simulink model "stm32test"  (R2024b)
settings: Solver=FixedStepAuto  StartTime=0.0  StopTime=inf  RelTol=1e-3  EnableMultiTasking=on
libraries: stm32f4xxblockslib x17, simulink x14, dspstat3 x2, stm32blockslib x2, simulink_extras x2, Blokk_Konyvtar x1
settings Model: STM32="{\"DigitalPortRead\":[{\"ID\":\"stm32test:431\"},{\"ID\":\"stm32test:432\"},{\"ID\":\"stm32test:483\"},{\"ID\":\"stm32test:484\"},{\"ID\":\"stm32test:504\"},{\"ID\":\"stm32test:505\"},{\"ID\":\"stm32test:895\"},{\"ID\":\"stm32test:896\"},{\"ID\":\"stm32test:1060\"},{\"ID\":\"stm32test:1031\"},{\"ID\":\"stm32test:1185\"},{\"ID\":\"stm32test:1186\"},{\"ID\":\"stm32test:1192\"},{\"ID\":\"stm32test:1193\"},{\"ID\":\"stm32test:1194\"},{\"ID\":\"stm32test:1195\"},{\"ID\":\"stm32test:1388:438\"},{\"ID\":\"stm32test:1424\"},{\"ID\":\"stm32test:1590\"}],\"PWMOutput\":[{\"ID\":\"stm32test:6\"},{\"ID\":\"stm32test:8\"},{\"ID\":\"stm32test:1305\"},{\"ID\":\"stm32test:1306\"},{\"ID\":\"stm32test:1562\"}],\"DigitalPortWrite\":[{\"ID\":\"stm32test:1295\"},{\"ID\":\"stm32test:1307\"},{\"ID\":\"stm32test:1481\"},{\"ID\":\"stm32test:1482\"}],\"TimerCapture\":[{\"ID\":\"stm32test:166\"},{\"ID\":\"stm32test:836\"},{\"ID\":\"stm32test:1074\"},{\"ID\":\"stm32test:1045\"},{\"ID\":\"stm32test:1103\"},{\"ID\":\"stm32test:1388:414\"},{\"ID\":\"stm32test:1132\"},{\"ID\":\"stm32test:1468:414\"},{\"ID\":\"stm32test:1542\"}],\"HardwareInterrupt\":[{\"ID\":\"stm32test:102\"},{\"ID\":\"stm32test:1388:418\"}]}"  Creator=Tarsoly  LastModifiedBy=Asus
settings OptimizationCC: BlockReduction=off  BooleanDataType=off  EnhancedBackFolding=on  PassReuseOutputArgsAs=Individual arguments  ZeroExternalMemoryAtStartup=off  ZeroInternalMemoryAtStartup=off  MaxStackSize=512  OptimizeBlockOrder=speed  DifferentSizesBufferReuse=on  OptimizationCustomize=off  EfficientTunableParamExpr=on
settings DebuggingCC: SaveWithParameterizedLinksMsg=none  MergeDetectMultiDrivingBlocksExec=none  SignalResolutionControl=TryResolveAllWithWarning  ParameterTunabilityLossMsg=error
settings HardwareCC: ProdBitPerPointer=32  ProdBitPerSizeT=32  ProdBitPerPtrDiffT=32  ProdLargestAtomicInteger=Long  ProdLargestAtomicFloat=Double  ProdWordSize=32  ProdHWDeviceType=ARM Compatible->ARM Cortex-M  TargetLargestAtomicInteger=Long  TargetLargestAtomicFloat=Double  TargetIntDivRoundTo=Zero  TargetEndianess=LittleEndian  TargetHWDeviceType=ARM Compatible->ARM Cortex-M
settings ModelReferenceCC: PropagateSignalLabelsOutOfModel=off
settings SFSimCC: SimCustomHeaderCode="#include \"SensorActuator.h\""  SimCustomInitializer=Timer_Init_Custom();  SimUserSources=SensorActuator.c  SimUserDefines=STM32F411xE  MATLABDynamicMemAlloc=off
settings SFSimCC: SimUserIncludeDirs=|
  | D:\BME\Hetedik_felev\Szakdoga\Matlab\C_kod
  | D:\CubeMXProjectFiles\tanfolyamrobot\Core\Inc
  | D:\CubeMXProjectFiles\tanfolyamrobot\Drivers\STM32F4xx_HAL_Driver\Inc
  | D:\CubeMXProjectFiles\tanfolyamrobot\Drivers\CMSIS\Device\ST\STM32F4xx\Include
  | D:\CubeMXProjectFiles\tanfolyamrobot\Drivers\CMSIS\Include
settings RTWCC: Description=Embedded Coder  SystemTargetFile=ert.tlc  HardwareBoard=STM32F4xx Based  TemplateMakefile=ert_default_tmf  RTWUseSimCustomCode=on  CustomHeaderCode="#include \"SensorActuator.h\""  CustomSource=SensorActuator.c  CustomDefine=STM32F411xE  CustomInitializer=Timer_Init_Custom();  Toolchain=GNU Tools for ARM Embedded Processors
settings RTWCC: CustomInclude=|
  | D:\BME\Hetedik_felev\Szakdoga\Matlab\C_kod
  | D:\CubeMXProjectFiles\tanfolyamrobot\Core\Inc
  | D:\CubeMXProjectFiles\tanfolyamrobot\Drivers\STM32F4xx_HAL_Driver\Inc
  | D:\CubeMXProjectFiles\tanfolyamrobot\Drivers\CMSIS\Device\ST\STM32F4xx\Include
  | D:\CubeMXProjectFiles\tanfolyamrobot\Drivers\CMSIS\Include
settings CodeAppCC: ForceParamTrailComments=on  IgnoreCustomStorageClasses=off  OperatorAnnotations=on  SimulinkDataObjDesc=on  SFDataObjDesc=on  InsertBlockDesc=on
settings ERTTargetCC: TargetLangStandard=C99 (ISO)  CodeReplacementLibrary=ARM Cortex-M  ExtModeTransport=3  ExtModeStaticAlloc=on  ExtModeStaticAllocSize=2048  ExtModeMexFile=ext_xcp  ExtModeIntrfLevel=Level2 - Open  InlinedParameterPlacement=Hierarchical

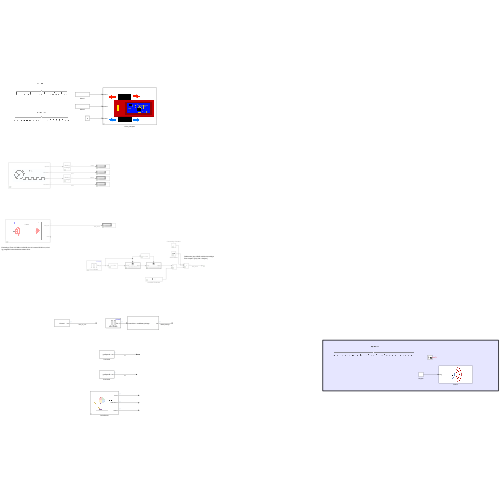
[thumbnail: Simulink's stored preview of the top-level diagram]
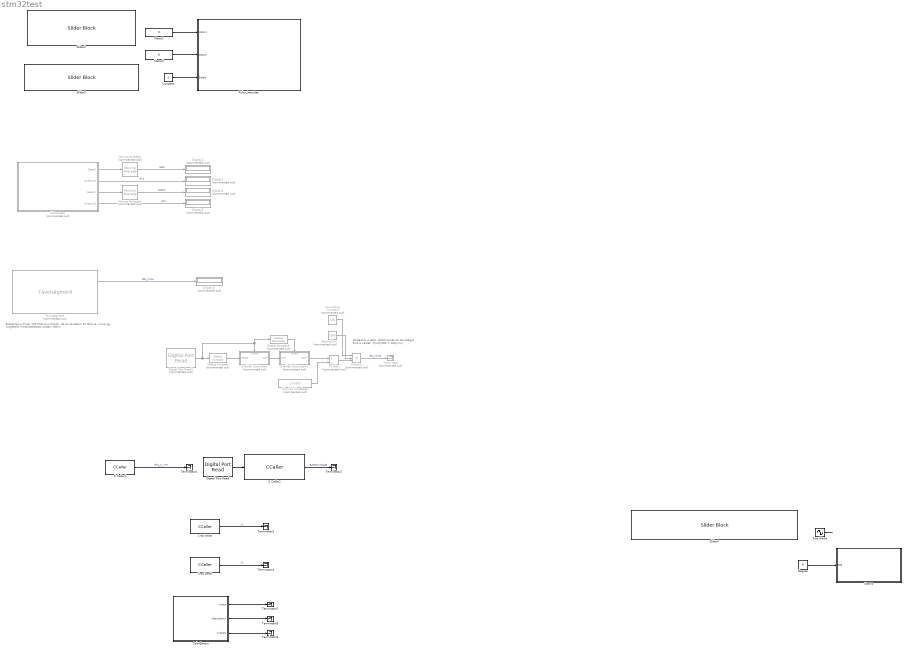
== system stm32test ==
  note: Eredetileg a Timer 100 MHz-el működik, de én levettem 25 MHz-re, mivel
      | így megfelelő mintavételezést tudtam elérni.
  note: Skálázzuk a jelet, időből csinálunk távolságot
      | Erra a képlet: T[ms]*100 = dist[mm]
  1-es kerek : CCaller  FunctionName=getSpeedA  PortSpecificationStruct="%)30     .    & (   8    (     @         %    \"     $    !     0         %  0 \"0    $    _    07)G3F%M90  4&]R=$YA;64 4V-O<&4     26YD97@     5'EP90      4VEZ90      27-';&]B86P   X    P    !@    @    $          4    (     0    ,    !         !   P!O=70 #@   #     &    \"     0         !0    @    !     P    $         $  # &]U=  .    .     8    (    !          %    \"     $    &     0         0    !@   $]U='!U=   #@   #@    &    \"     8         !0    @    !     0    $         \"0    @               X    X    !@    @    $          4    (     0    8    !         !     &    9&]U8FQE   .    ,     8    (    !          %    \"     $    !     0         0  $ ,0    X    P    !@    @    ) @        4    (     0    $    !          (  0"  SampleTime=0.02
  2-es kerek : CCaller  FunctionName=getSpeedB  PortSpecificationStruct="%)30     .    & (   8    (     @         %    \"     $    !     0         %  0 \"0    $    _    07)G3F%M90  4&]R=$YA;64 4V-O<&4     26YD97@     5'EP90      4VEZ90      27-';&]B86P   X    P    !@    @    $          4    (     0    ,    !         !   P!O=70 #@   #     &    \"     0         !0    @    !     P    $         $  # &]U=  .    .     8    (    !          %    \"     $    &     0         0    !@   $]U='!U=   #@   #@    &    \"     8         !0    @    !     0    $         \"0    @               X    X    !@    @    $          4    (     0    8    !         !     &    9&]U8FQE   .    ,     8    (    !          %    \"     $    !     0         0  $ ,0    X    P    !@    @    ) @        4    (     0    $    !          (  0"  SampleTime=0.02
  C Caller1 : CCaller  FunctionName=infrared  PortSpecificationStruct="%)30     .    & (   8    (     @         %    \"     $    !     0         %  0 \"0    $    _    07)G3F%M90  4&]R=$YA;64 4V-O<&4     26YD97@     5'EP90      4VEZ90      27-';&]B86P   X    P    !@    @    $          4    (     0    ,    !         !   P!O=70 #@   #     &    \"     0         !0    @    !     P    $         $  # &]U=  .    .     8    (    !          %    \"     $    &     0         0    !@   $]U='!U=   #@   #@    &    \"     8         !0    @    !     0    $         \"0    @               X    X    !@    @    $          4    (     0    8    !         !     &    =6EN=#,R   .    ,     8    (    !          %    \"     $    !     0         0  $ ,0    X    P    !@    @    ) @        4    (     0    $    !          (  0"  SampleTime=0.02
  C Caller2 : CCaller  FunctionName=readBatteryVoltage  PortSpecificationStruct="%)30     .    V ,   8    (     @         %    \"     (    !     0         %  0 \"0    $    _    07)G3F%M90  4&]R=$YA;64 4V-O<&4     26YD97@     5'EP90      4VEZ90      27-';&]B86P   X    P    !@    @    $          4    (     0    ,    !         !   P!O=70 #@   #     &    \"     0         !0    @    !     P    $         $  # &]U=  .    .     8    (    !          %    \"     $    &     0         0    !@   $]U='!U=   #@   #@    &    \"     8         !0    @    !     0    $         \"0    @               X    X    !@    @    $          4    (     0    8    !         !     &    =6EN=#$V   .    ,     8    (    !          %    \"     $    !     0         0  $ ,0    X    P    !@    @    ) @        4    (     0    $    !          (  0      #@   $     &    \"     0         !0    @    !    \"P    $         $     L   !B=71T;VY686QU90      #@   $     &    \"     0         !0    @    !    \"P    $         $     L   !B=71T;VY686QU90      #@   #@    &    \"     0         !0    @    !    !0    $         $     4   !);G!U=     X    X    !@    @    &          4    (     0    $    !          D    (               .    .     8    (    !          %    \"     $    '     0         0    !P   &)O;VQE86X #@   #     &    \"     0         !0    @    !     0    $         $  ! #$    .    ,     8    (    \"0(        %    \"     $    !     0         \"  $"  SampleTime=1
  ColorSensor : Subsystem
      mask DialogControl DescTextVar Prompt: This subsystem is for measuring the color of the ground beneath the robot.
      mask Display: image('Mask5_szin2.png', [20,20,20,20,100,100]);
  Constant : Constant
  Converting Constant : Constant  Commented=on  Value=100
  Degree : Constant  Value=0
  Detect Decrease : simulink/Logic and Bit Operations/Detect Decrease  Commented=on  vinit=0.0  OutDataTypeStr=boolean
  Detect Increase : simulink/Logic and Bit Operations/Detect Increase  Commented=on  vinit=0.0  OutDataTypeStr=boolean
  Digital Port Read : stm32f4xxblockslib/Digital Port Read  PortName=GPIOA  PinNumber=[15]  ReadOperation=on  IOAsArray=off  SampleTime=1  EnableSimPort=off  hoistedMaskSrc=ECSoC/ECSimCodegen/Digital Port Read
  Digital Port Read1 : stm32f4xxblockslib/Digital Port Read  Commented=on  PortName=GPIOB  PinNumber=[7]  ReadOperation=on  IOAsArray=on  SampleTime=0.0001  EnableSimPort=off  hoistedMaskSrc=ECSoC/ECSimCodegen/Digital Port Read
  Display{1..4,6} (5 alike) : Display  Commented=on
  Divide1 : Product  Commented=on  Inputs=*/
  Enabled Subsystem : Subsystem  Commented=on  TreatAsAtomicUnit=on
  Enabled Subsystem1 : Subsystem  Commented=on  TreatAsAtomicUnit=on
  Kulon_iranyitas : Subsystem
      mask DialogControl Control2 Prompt: This block is meant for when you want to control the wheels independent of eachother. It can control the wheels with (-99;99) signals.
      mask Display: image('Maszk4_kulon_kerek.png', [25,25,5,0,100,100]);
  Motor1 : Constant  Value=0
  Motor2 : Constant  Value=0
  Moving Average : dspstat3/Moving Average  Commented=on  Method=Sliding window  ForgettingFactorPort=off  SpecifyWindowLength=on  WindowLength=5  OverlapLength=4  AllowArbitraryInputLength=off  ForgettingFactor=0.9  SimulateUsing=Interpreted execution
  Moving Average1 : dspstat3/Moving Average  Commented=on  Method=Sliding window  ForgettingFactorPort=off  SpecifyWindowLength=on  WindowLength=9  OverlapLength=8  AllowArbitraryInputLength=off  ForgettingFactor=0.9  SimulateUsing=Interpreted execution
  Product : Product  Commented=on  Inputs=3
  Second2ms : Constant  Commented=on  Value=1000
  Simulink Timebase : Constant  Commented=on  Value=1/0.0001
  Sine Wave : Sin  Amplitude=90  Frequency=pi  SampleTime=0.02
  Slider2 : SliderBlock  ScaleMin=-99  ScaleMax=99
  Slider3 : SliderBlock  ScaleMin=-99  ScaleMax=99
  Slider4 : SliderBlock  ScaleMin=-90  ScaleMax=90
  Subsystem : Subsystem  Commented=on  mask{TimClkFrq=25e6, CPR=1024, fwdvalue1=0, fwdvalue2=1, bckvalue1=1, bckvalue2=0, PrScaler=1}
      mask prompts: TimClkFrq "Timer Clock Frequency"; CPR "Counts Per Revolution"; fwdvalue1 "Forward Direction Value 1"; fwdvalue2 "Forward Direction Value 2"; bckvalue1 "Backward Direction Value 1"; bckvalue2 "Backward Direction Value 2"; PrScaler "Timer Prescaler (Shouldn't be Zero)"
      mask DialogControl DescTextVar Prompt: This block takes the encoder signal and converts it into speed and direction. The frequency of the timer channel and the counts per revolution is required to be filled with the correct values. The direction signals for each wheel is also customisable, thus the wheels may have a different base direction. The block uses Timer5 hardware interrupt on all 4 channels and reads PA0-3 GPIO ports. Modifying this requires looking under the mask.
      mask Display: image('Mask1.png', [30,10,30,10,100,100]);
  Szervo : Subsystem
      mask Display: image('Mask6_Szervo.png', [30,10,30,10,100,100]);
  Terminator : Terminator  Commented=on
  Terminator{1..7} (7 alike) : Terminator
  Távolságmérő : Blokk_Konyvtar/Távolságmérő  Commented=on  TimClkFrq=25e6  PrScaler=15000  OoR_const=2000
      settings: SourceProductName=Blokk_Konyvtar
  wires:
  Moving Average/1 -> Display2/1  "rad/s"
  Moving Average1/1 -> Display4/1  "rad/s2"
  Távolságmérő/1 -> Display6/1  "dist_mma"
  Subsystem/1(Speed1) -> Moving Average/1
  Subsystem/2(Direction1) -> Display1/1  "dir1"
  Subsystem/3(Speed 2) -> Moving Average1/1
  Subsystem/4(Direction2) -> Display3/1  "dir2"
  Constant/1 -> Kulon_iranyitas/3(Enable)
  Motor1/1 -> Kulon_iranyitas/1(Motor1)
  Motor2/1 -> Kulon_iranyitas/2(Motor2)
  Digital Port Read1/1 -> Detect Increase/1, Detect Decrease/1, Enabled Subsystem/Enable
  Detect Increase/1 -> Enabled Subsystem/1(Reset)
  Enabled Subsystem/1(CNT) -> Enabled Subsystem1/1(CNT)
  Detect Decrease/1 -> Enabled Subsystem1/Enable
  Second2ms/1 -> Product/2
  Enabled Subsystem1/1(Latch) -> Divide1/1
  Converting Constant/1 -> Product/1
  Simulink Timebase/1 -> Divide1/2
  Divide1/1 -> Product/3
  Product/1 -> Terminator/1  "dist_mmb"
  C Caller1/1 -> Terminator1/1  "Infra_C_mm"
  C Caller2/1 -> Terminator2/1  "BatteryVoltage"
  Digital Port Read/1 -> C Caller2/1
  2-es kerek/1 -> Terminator4/1  "v2"
  1-es kerek/1 -> Terminator3/1  "v1"
  Sine Wave/1 -> ?
  ColorSensor/1(<Hue>) -> Terminator7/1
  ColorSensor/2(<Saturation>) -> Terminator5/1
  ColorSensor/3(<Value>) -> Terminator6/1
  Degree/1 -> Szervo/1(Deg)

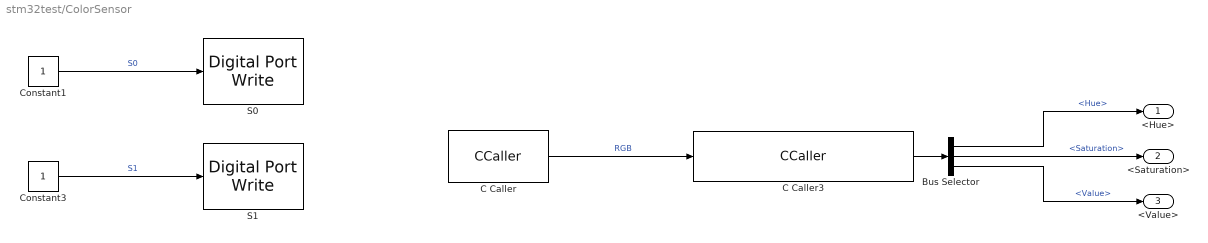
== system stm32test/ColorSensor ==
  Bus Selector : BusSelector  OutputSignals=Hue,Saturation,Value
  C Caller : CCaller  FunctionName=getRGB  PortSpecificationStruct="%)30     .    ( (   8    (     @         %    \"     $    !     0         %  0 \"0    $    _    07)G3F%M90  4&]R=$YA;64 4V-O<&4     26YD97@     5'EP90      4VEZ90      27-';&]B86P   X    P    !@    @    $          4    (     0    ,    !         !   P!O=70 #@   #     &    \"     0         !0    @    !     P    $         $  # &]U=  .    .     8    (    !          %    \"     $    &     0         0    !@   $]U='!U=   #@   #@    &    \"     8         !0    @    !     0    $         \"0    @               X   !     !@    @    $          4    (     0    H    !         !     *    0G5S.B!21T)?=         X    P    !@    @    $          4    (     0    $    !         !   0 Q    #@   #     &    \"     D\"        !0    @    !     0    $          @ !"  SampleTime=0.02
  C Caller3 : CCaller  FunctionName=getHSVfromRGB  PortSpecificationStruct="%)30     .    Z ,   8    (     @         %    \"     (    !     0         %  0 \"0    $    _    07)G3F%M90  4&]R=$YA;64 4V-O<&4     26YD97@     5'EP90      4VEZ90      27-';&]B86P   X    P    !@    @    $          4    (     0    ,    !         !   P!O=70 #@   #     &    \"     0         !0    @    !     P    $         $  # &]U=  .    .     8    (    !          %    \"     $    &     0         0    !@   $]U='!U=   #@   #@    &    \"     8         !0    @    !     0    $         \"0    @               X   !     !@    @    $          4    (     0    H    !         !     *    0G5S.B!(4U9?=         X    P    !@    @    $          4    (     0    $    !         !   0 Q    #@   #     &    \"     D\"        !0    @    !     0    $          @ !       .    0     8    (    !          %    \"     $    +     0         0    \"P   &UE87-U<F5M96YT       .    0     8    (    !          %    \"     $    +     0         0    \"P   &UE87-U<F5M96YT       .    .     8    (    !          %    \"     $    %     0         0    !0   $EN<'5T    #@   #@    &    \"     8         !0    @    !     0    $         \"0    @               X   !     !@    @    $          4    (     0    H    !         !     *    0G5S.B!21T)?=         X    P    !@    @    $          4    (     0    $    !         !   0 Q    #@   #     &    \"     D\"        !0    @    !     0    $          @ !"
  Constant1 : Constant
  Constant3 : Constant
  S0 : stm32f4xxblockslib/Digital Port Write  PortName=GPIOC  PinNumber=[12]  ReadOperation=off  IOAsArray=on  EnableSimPort=off  hoistedMaskSrc=ECSoC/ECSimCodegen/Digital Port Write
  S1 : stm32f4xxblockslib/Digital Port Write  PortName=GPIOD  PinNumber=[2]  ReadOperation=off  IOAsArray=on  EnableSimPort=off  hoistedMaskSrc=ECSoC/ECSimCodegen/Digital Port Write
  <Hue> : Outport
  <Saturation> : Outport  Port=2
  <Value> : Outport  Port=3
  wires:
  C Caller/1 -> C Caller3/1  "RGB"
  Constant3/1 -> S1/1  "S1"
  Bus Selector/3 -> <Value>/1  "<Value>"
  C Caller3/1 -> Bus Selector/1
  Constant1/1 -> S0/1  "S0"
  Bus Selector/2 -> <Saturation>/1  "<Saturation>"
  Bus Selector/1 -> <Hue>/1  "<Hue>"

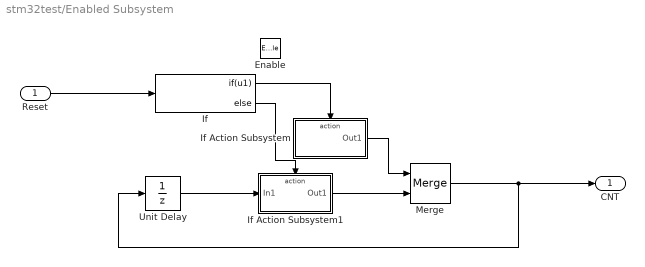
== system stm32test/Enabled Subsystem ==
  Reset : Inport
  Enable : EnablePort
  If : If  IfExpression=u1
  If Action Subsystem : Subsystem  TreatAsAtomicUnit=on
  If Action Subsystem1 : Subsystem  TreatAsAtomicUnit=on
  Merge : Merge
  Unit Delay : UnitDelay  SampleTime=-1  HasFrameUpgradeWarning=on
  CNT : Outport
  wires:
  Merge/1 -> Unit Delay/1, CNT/1
  Reset/1 -> If/1
  If/1 -> If Action Subsystem/Action
  If Action Subsystem/1(Out1) -> Merge/1
  If/2 -> If Action Subsystem1/Action
  If Action Subsystem1/1(Out1) -> Merge/2
  Unit Delay/1 -> If Action Subsystem1/1(In1)

== system stm32test/Enabled Subsystem1 ==
  CNT : Inport
  Enable : EnablePort
  Latch : Outport
  wires:
  CNT/1 -> Latch/1

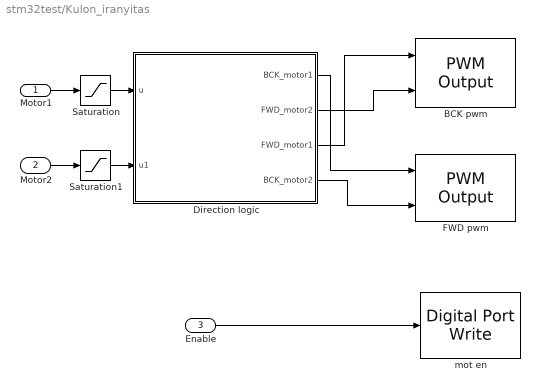
== system stm32test/Kulon_iranyitas ==
  Motor1 : Inport
  Motor2 : Inport  Port=2
  Enable : Inport  Port=3
  BCK pwm : stm32f4xxblockslib/PWM Output  TimerModule=TIM1  DutycycleUnits=Percentage  EnableChannel1=on  EnableChannel2=on  EnableChannel3=off  EnableChannel4=off  EnableCounterInput=off  EnableMainOutputInput=off  EnableFrequencyInput=off  SetRCAfterCE=off  OutputDirection=off  OutputMainOutputEnableStatus=off  SampleTime=0.1  EnableSimPort=off  EnableUpdateEvent=off  EnableCaptureCompare1Event=off  EnableCaptureCompare2Event=off  EnableCaptureCompare3Event=off  EnableCaptureCompare4Event=off  EnableTriggerEvent=off  EnableBreakEvent=off  ProcessorFamily=STM32F4  hoistedMaskSrc=ECSoC/ECSimCodegen/PWM Output
  Direction logic : Subsystem
  "FWD pwm " : stm32f4xxblockslib/PWM Output  TimerModule=TIM3  DutycycleUnits=Percentage  EnableChannel1=off  EnableChannel2=off  EnableChannel3=on  EnableChannel4=on  EnableCounterInput=off  EnableMainOutputInput=off  EnableFrequencyInput=off  SetRCAfterCE=off  OutputDirection=off  OutputMainOutputEnableStatus=off  SampleTime=0.1  EnableSimPort=off  EnableUpdateEvent=off  EnableCaptureCompare1Event=off  EnableCaptureCompare2Event=off  EnableCaptureCompare3Event=off  EnableCaptureCompare4Event=off  EnableTriggerEvent=off  EnableBreakEvent=off  ProcessorFamily=STM32F4  hoistedMaskSrc=ECSoC/ECSimCodegen/PWM Output
  Saturation : Saturate  UpperLimit=99  LowerLimit=-99
  Saturation1 : Saturate  UpperLimit=99  LowerLimit=-99
  mot en : stm32f4xxblockslib/Digital Port Write  PortName=GPIOC  PinNumber=5  ReadOperation=off  IOAsArray=on  EnableSimPort=off  hoistedMaskSrc=ECSoC/ECSimCodegen/Digital Port Write
  wires:
  Enable/1 -> mot en/1
  Motor1/1 -> Saturation/1
  Motor2/1 -> Saturation1/1
  Direction logic/1(BCK_motor1) -> "FWD pwm "/1
  Direction logic/2(FWD_motor2) -> BCK pwm/2
  Direction logic/3(FWD_motor1) -> BCK pwm/1
  Direction logic/4(BCK_motor2) -> "FWD pwm "/2
  Saturation/1 -> Direction logic/1(u)
  Saturation1/1 -> Direction logic/2(u1)

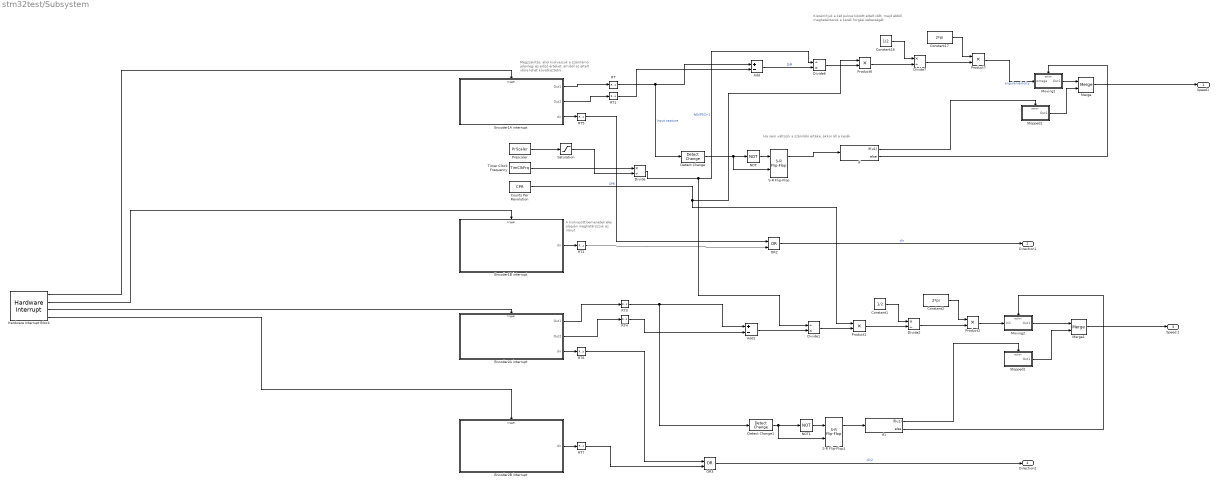
== system stm32test/Subsystem ==
  note: Kiszámítjuk a két pulzus között eltelt időt, majd ebből meghatározzuk a kerék forgási sebességét
  note: Ha nem változik a számláló értéke, akkor áll a kerék
  note: A kiolvasott bemenetek élei alapján meghatározzuk az irányt
  note: Megszakítás, ahol kiolvassuk a számlámó jelenlegi és előző értéket, amiből az eltelt időre lehet következtetni
  Add : Sum  Inputs=+-
  Add1 : Sum  Inputs=+-
  Constant1 : Constant  Value=1/2
  Constant16 : Constant  Value=1/2
  Constant17 : Constant  Value=2*pi
  Constant2 : Constant  Value=2*pi
  Counts Per Revolution : Constant  Value=CPR
  Detect Change : simulink/Logic and Bit Operations/Detect Change  vinit=0  OutDataTypeStr=boolean
      settings: LibrarySourceBlock=|
      | hdlsllib/Logic and Bit
      | Operations/Detect
      | Change
  Detect Change1 : simulink/Logic and Bit Operations/Detect Change  vinit=0  OutDataTypeStr=boolean
      settings: LibrarySourceBlock=|
      | hdlsllib/Logic and Bit
      | Operations/Detect
      | Change
  Divide : Product  Inputs=*/
  Divide1 : Product  Inputs=/*
  Divide2 : Product  Inputs=*/
  Divide6 : Product  Inputs=/*
  Divide7 : Product  Inputs=*/
  Encoder1A interrupt : Subsystem  TreatAsAtomicUnit=on
  Encoder1B interrupt : Subsystem  TreatAsAtomicUnit=on
  Encoder2A interrupt : Subsystem  TreatAsAtomicUnit=on
  Encoder2B interrupt : Subsystem  TreatAsAtomicUnit=on
  Hardware Interrupt Block : stm32f4xxblockslib/Hardware Interrupt  ISRGroup=Timer (TIM)  ISRName=TIM5_IRQHandler  ISRNumber=65  EventsList={ 'off', 'TIM5 Update', '1'; 'on', 'TIM5 CC1', '2'; 'on', 'TIM5 CC2', '3'; 'on', 'TIM5 CC3', '4'; 'on', 'TIM5 CC4', '5'; 'off', 'TIM5 Trigger', '6'; 'off', 'Custom event', '7' }  SelectedEvents={'TIM5 CC1','TIM5 CC2','TIM5 CC3','TIM5 CC4'}  TaskPriority=30  DisablePreemption=off  ClearInterruptFlagsAtEndOfEvent=on  InterruptDefinitionFile=$(TARGET_ROOT)/registry/interrupts/STM32F4xxBased_interrupts.xml  HardwareBoard=STM32F4xx Based  EnableSimPort=off
  If : If  IfExpression=u1
  If1 : If  IfExpression=u1
  Merge : Merge
  Merge1 : Merge
  Moving1 : Subsystem  TreatAsAtomicUnit=on
  Moving2 : Subsystem  TreatAsAtomicUnit=on
  NOT : Logic  Operator=NOT  IconShape=distinctive  AllPortsSameDT=off  OutDataTypeStr=boolean
  NOT1 : Logic  Operator=NOT  IconShape=distinctive  AllPortsSameDT=off  OutDataTypeStr=boolean
  OR2 : Logic  Operator=OR  IconShape=distinctive  AllPortsSameDT=off  OutDataTypeStr=boolean
  OR3 : Logic  Operator=OR  IconShape=distinctive  AllPortsSameDT=off  OutDataTypeStr=boolean
  Prescaler : Constant  Value=PrScaler
  Product{1..2,6..7} (4 alike) : Product
  RT{,1..7} (8 alike) : RateTransition  Deterministic=off  OutPortSampleTime=0.02
  S-R Flip-Flop : simulink_extras/Flip Flops/S-R Flip-Flop  initial_condition=0
  S-R Flip-Flop1 : simulink_extras/Flip Flops/S-R Flip-Flop  initial_condition=0
  Saturation : Saturate  UpperLimit=inf  LowerLimit=1
  Stopped1 : Subsystem  TreatAsAtomicUnit=on
  Stopped2 : Subsystem  TreatAsAtomicUnit=on
  Timer Clock Frequency : Constant  Value=TimClkFrq
  Speed1 : Outport
  Direction1 : Outport  Port=2
  Speed 2 : Outport  Port=3
  Direction2 : Outport  Port=4
  wires:
  S-R Flip-Flop1/1 -> If1/1
  Hardware Interrupt Block/4 -> Encoder2B interrupt/Trigger
  Encoder1A interrupt/2(Out2) -> RT1/1
  Product7/1 -> Moving1/1(omega)  "angularvelocity"
  Stopped2/1(Out1) -> Merge1/2
  If/1 -> Stopped1/Action
  Moving1/1(Out1) -> Merge/1
  RT6/1 -> OR3/1
  If/2 -> Moving1/Action
  Hardware Interrupt Block/2 -> Encoder1B interrupt/Trigger
  Detect Change1/1 -> NOT1/1, S-R Flip-Flop1/2
  Hardware Interrupt Block/1 -> Encoder1A interrupt/Trigger
  Encoder2A interrupt/1(Out1) -> RT3/1
  If1/1 -> Stopped2/Action
  OR3/1 -> Direction2/1  "dir2"
  NOT/1 -> S-R Flip-Flop/1
  RT4/1 -> Add1/2
  Encoder2A interrupt/2(Out2) -> RT4/1
  Encoder1A interrupt/1(Out1) -> RT/1
  S-R Flip-Flop/1 -> If/1
  RT7/1 -> OR3/2
  Moving2/1(Out1) -> Merge1/1
  Hardware Interrupt Block/3 -> Encoder2A interrupt/Trigger
  If1/2 -> Moving2/Action
  RT/1 -> Add/1, Detect Change/1  "Input capture"
  Stopped1/1(Out1) -> Merge/2
  RT3/1 -> Add1/1, Detect Change1/1
  RT5/1 -> OR2/1
  RT2/1 -> OR2/2
  NOT1/1 -> S-R Flip-Flop1/1
  Merge1/1 -> Speed 2/1
  Detect Change/1 -> NOT/1, S-R Flip-Flop/2
  Merge/1 -> Speed1/1
  RT1/1 -> Add/2
  Product2/1 -> Moving2/1(In1)
  OR2/1 -> Direction1/1  "dir"
  Encoder1B interrupt/1(dir) -> RT2/1
  Encoder1A interrupt/3(dir) -> RT5/1
  Encoder2A interrupt/3(dir) -> RT6/1
  Encoder2B interrupt/1(dir) -> RT7/1
  Timer Clock Frequency/1 -> Divide/1
  Prescaler/1 -> Saturation/1
  Divide/1 -> Divide6/1, Divide1/1  "fclk/PSC+1"
  Counts Per Revolution/1 -> Product1/1, Product6/1  "CPR"
  Product6/1 -> Divide7/2
  Divide7/1 -> Product7/2
  Divide6/1 -> Product6/2
  Add/1 -> Divide6/2  "Diff"
  Constant17/1 -> Product7/1
  Constant16/1 -> Divide7/1
  Saturation/1 -> Divide/2
  Divide1/1 -> Product1/2
  Add1/1 -> Divide1/2
  Constant1/1 -> Divide2/1
  Product1/1 -> Divide2/2
  Divide2/1 -> Product2/2
  Constant2/1 -> Product2/1

== system stm32test/Szervo ==
  Deg : Inport
  PWM Output : stm32f4xxblockslib/PWM Output  TimerModule=TIM11  DutycycleUnits=Percentage  EnableChannel1=on  EnableChannel2=off  EnableChannel3=off  EnableChannel4=off  EnableCounterInput=off  EnableMainOutputInput=off  EnableFrequencyInput=off  SetRCAfterCE=off  OutputDirection=off  OutputMainOutputEnableStatus=off  SampleTime=0.1  EnableSimPort=off  EnableUpdateEvent=off  EnableCaptureCompare1Event=off  EnableCaptureCompare2Event=off  EnableCaptureCompare3Event=off  EnableCaptureCompare4Event=off  EnableTriggerEvent=off  EnableBreakEvent=off  ProcessorFamily=STM32F4  hoistedMaskSrc=ECSoC/ECSimCodegen/PWM Output
  Subsystem2 : Subsystem
  wires:
  Subsystem2/1(f(x)) -> PWM Output/1  "percent"
  Deg/1 -> Subsystem2/1(x)  "x"

== system stm32test/Enabled Subsystem/If Action Subsystem ==
  Action Port : ActionPort  ActionPortLabel=if(u1)
  Constant : Constant  Value=0
  Out1 : Outport
  wires:
  Constant/1 -> Out1/1

== system stm32test/Enabled Subsystem/If Action Subsystem1 ==
  In1 : Inport
  Action Port : ActionPort  ActionPortLabel=else
  Add Constant : Bias  Bias=1  SaturateOnIntegerOverflow=off
  Out1 : Outport
  wires:
  Add Constant/1 -> Out1/1
  In1/1 -> Add Constant/1

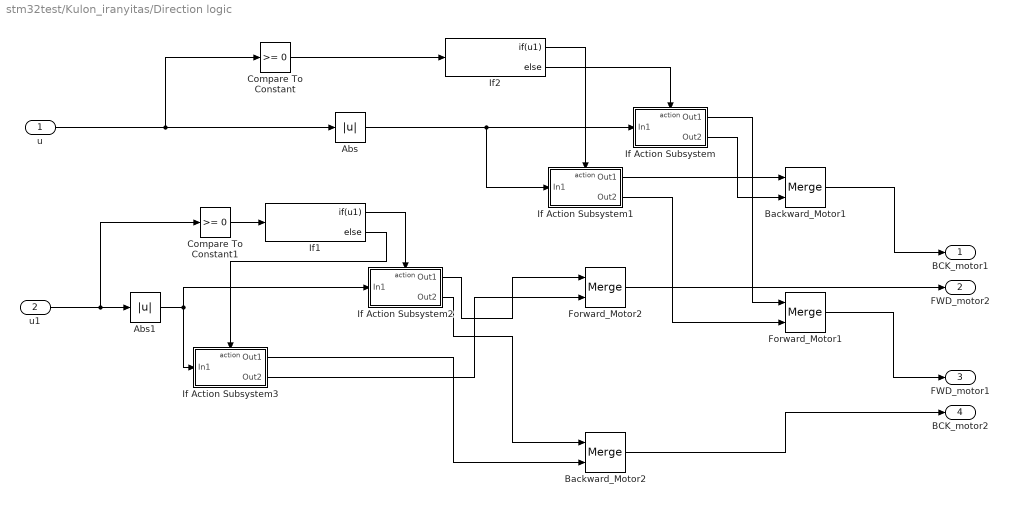
== system stm32test/Kulon_iranyitas/Direction logic ==
  u : Inport
  u1 : Inport  Port=2
  Abs : Abs  SaturateOnIntegerOverflow=off
  Abs1 : Abs  SaturateOnIntegerOverflow=off
  Backward_Motor1 : Merge
  Backward_Motor2 : Merge
  Compare To Constant : simulink/Logic and Bit Operations/Compare To Constant  relop=>=  const=0  OutDataTypeStr=boolean
  Compare To Constant1 : simulink/Logic and Bit Operations/Compare To Constant  relop=>=  const=0  OutDataTypeStr=boolean
  Forward_Motor1 : Merge
  Forward_Motor2 : Merge
  If Action Subsystem : Subsystem  TreatAsAtomicUnit=on
  If Action Subsystem1 : Subsystem  TreatAsAtomicUnit=on
  If Action Subsystem2 : Subsystem  TreatAsAtomicUnit=on
  If Action Subsystem3 : Subsystem  TreatAsAtomicUnit=on
  If1 : If  IfExpression=u1
  If2 : If  IfExpression=u1
  BCK_motor1 : Outport
  FWD_motor2 : Outport  Port=2
  FWD_motor1 : Outport  Port=3
  BCK_motor2 : Outport  Port=4
  wires:
  Forward_Motor2/1 -> FWD_motor2/1
  If Action Subsystem/1(Out1) -> Forward_Motor1/1
  If Action Subsystem1/1(Out1) -> Backward_Motor1/1
  If Action Subsystem3/2(Out2) -> Forward_Motor2/2
  Compare To Constant/1 -> If2/1
  If Action Subsystem3/1(Out1) -> Backward_Motor2/2
  Abs1/1 -> If Action Subsystem2/1(In1), If Action Subsystem3/1(In1)
  Abs/1 -> If Action Subsystem1/1(In1), If Action Subsystem/1(In1)
  If Action Subsystem/2(Out2) -> Backward_Motor1/2
  u/1 -> Abs/1, Compare To Constant/1
  Backward_Motor2/1 -> BCK_motor2/1
  If1/1 -> If Action Subsystem2/Action
  Compare To Constant1/1 -> If1/1
  u1/1 -> Compare To Constant1/1, Abs1/1
  Backward_Motor1/1 -> BCK_motor1/1
  If1/2 -> If Action Subsystem3/Action
  If Action Subsystem1/2(Out2) -> Forward_Motor1/2
  If Action Subsystem2/1(Out1) -> Forward_Motor2/1
  If Action Subsystem2/2(Out2) -> Backward_Motor2/1
  Forward_Motor1/1 -> FWD_motor1/1
  If2/2 -> If Action Subsystem/Action
  If2/1 -> If Action Subsystem1/Action

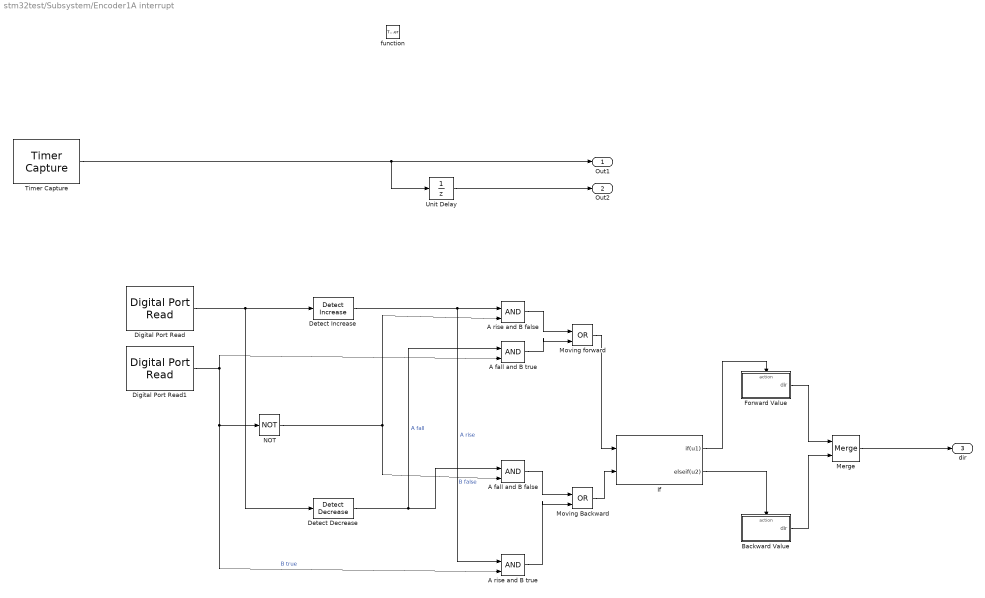
== system stm32test/Subsystem/Encoder1A interrupt ==
  function : TriggerPort  TriggerType=function-call  VariantControl=(inherit)
  A fall and B false : Logic  IconShape=distinctive  AllPortsSameDT=off  OutDataTypeStr=boolean
  A fall and B true : Logic  IconShape=distinctive  AllPortsSameDT=off  OutDataTypeStr=boolean
  A rise and B false : Logic  IconShape=distinctive  AllPortsSameDT=off  OutDataTypeStr=boolean
  A rise and B true : Logic  IconShape=distinctive  AllPortsSameDT=off  OutDataTypeStr=boolean
  Backward Value : Subsystem  TreatAsAtomicUnit=on
  Detect Decrease : simulink/Logic and Bit Operations/Detect Decrease  vinit=0.0  OutDataTypeStr=boolean
  Detect Increase : simulink/Logic and Bit Operations/Detect Increase  vinit=0.0  OutDataTypeStr=boolean
  Digital Port Read : stm32f4xxblockslib/Digital Port Read  PortName=GPIOA  PinNumber=[0]  ReadOperation=on  IOAsArray=on  SampleTime=-1  EnableSimPort=off  hoistedMaskSrc=ECSoC/ECSimCodegen/Digital Port Read
  Digital Port Read1 : stm32f4xxblockslib/Digital Port Read  PortName=GPIOA  PinNumber=[1]  ReadOperation=on  IOAsArray=on  SampleTime=-1  EnableSimPort=off  hoistedMaskSrc=ECSoC/ECSimCodegen/Digital Port Read
  Forward Value : Subsystem  TreatAsAtomicUnit=on
  If : If  NumInputs=2  IfExpression=u1  ElseIfExpressions=u2  ShowElse=off
  Merge : Merge
  Moving Backward : Logic  Operator=OR  IconShape=distinctive  AllPortsSameDT=off  OutDataTypeStr=boolean
  Moving forward : Logic  Operator=OR  IconShape=distinctive  AllPortsSameDT=off  OutDataTypeStr=boolean
  NOT : Logic  Operator=NOT  IconShape=distinctive  AllPortsSameDT=off  OutDataTypeStr=boolean
  Timer Capture : stm32blockslib/Timer Capture  TimerModule=TIM5  SelectedChannel=CH1  CaptureLength=1  OutputDataLength=off  OutputOverrunStatus=off  OutputDirection=off  SampleTime=-1
      settings: LibrarySourceBlock=stm32f4xxblockslib/Timer Capture
  Unit Delay : UnitDelay  SampleTime=-1  HasFrameUpgradeWarning=on
  Out1 : Outport
  Out2 : Outport  Port=2
  dir : Outport  Port=3
  wires:
  Timer Capture/1 -> Out1/1, Unit Delay/1
  Unit Delay/1 -> Out2/1
  If/2 -> Backward Value/Action
  A rise and B false/1 -> Moving forward/1
  A fall and B false/1 -> Moving Backward/1
  Moving forward/1 -> If/1
  A rise and B true/1 -> Moving Backward/2
  Forward Value/1(dir) -> Merge/1
  Digital Port Read/1 -> Detect Decrease/1, Detect Increase/1
  A fall and B true/1 -> Moving forward/2
  Digital Port Read1/1 -> A rise and B true/2, NOT/1, A fall and B true/2  "B true"
  Merge/1 -> dir/1
  Detect Increase/1 -> A rise and B true/1, A rise and B false/1  "A rise"
  NOT/1 -> A fall and B false/2, A rise and B false/2  "B false"
  Moving Backward/1 -> If/2
  Detect Decrease/1 -> A fall and B false/1, A fall and B true/1  "A fall"
  Backward Value/1(dir) -> Merge/2
  If/1 -> Forward Value/Action

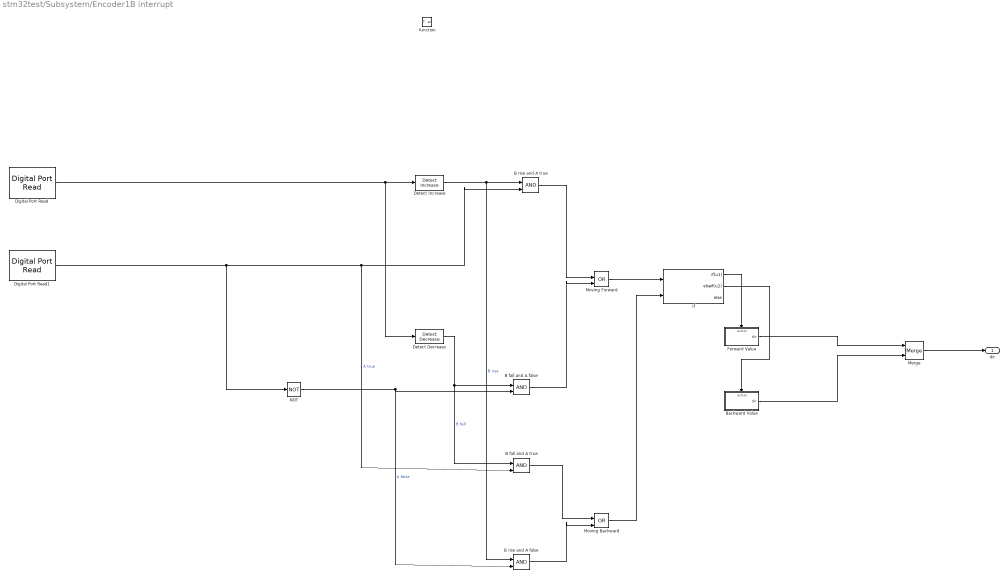
== system stm32test/Subsystem/Encoder1B interrupt ==
  function : TriggerPort  TriggerType=function-call  VariantControl=(inherit)
  B fall and A false : Logic  IconShape=distinctive  AllPortsSameDT=off  OutDataTypeStr=boolean
  B fall and A true : Logic  IconShape=distinctive  AllPortsSameDT=off  OutDataTypeStr=boolean
  B rise and A false : Logic  IconShape=distinctive  AllPortsSameDT=off  OutDataTypeStr=boolean
  B rise and A true : Logic  IconShape=distinctive  AllPortsSameDT=off  OutDataTypeStr=boolean
  Backward Value : Subsystem  TreatAsAtomicUnit=on
  Detect Decrease : simulink/Logic and Bit Operations/Detect Decrease  vinit=0.0  OutDataTypeStr=boolean
  Detect Increase : simulink/Logic and Bit Operations/Detect Increase  vinit=0.0  OutDataTypeStr=boolean
  Digital Port Read : stm32f4xxblockslib/Digital Port Read  PortName=GPIOA  PinNumber=[1]  ReadOperation=on  IOAsArray=on  SampleTime=-1  EnableSimPort=off  hoistedMaskSrc=ECSoC/ECSimCodegen/Digital Port Read
  Digital Port Read1 : stm32f4xxblockslib/Digital Port Read  PortName=GPIOA  PinNumber=[0]  ReadOperation=on  IOAsArray=on  SampleTime=-1  EnableSimPort=off  hoistedMaskSrc=ECSoC/ECSimCodegen/Digital Port Read
  Forward Value : Subsystem  TreatAsAtomicUnit=on
  If : If  NumInputs=2  IfExpression=u1  ElseIfExpressions=u2
  Merge : Merge
  Moving Backward : Logic  Operator=OR  IconShape=distinctive  AllPortsSameDT=off  OutDataTypeStr=boolean
  Moving Forward : Logic  Operator=OR  IconShape=distinctive  AllPortsSameDT=off  OutDataTypeStr=boolean
  NOT : Logic  Operator=NOT  IconShape=distinctive  AllPortsSameDT=off  OutDataTypeStr=boolean
  dir : Outport
  wires:
  Digital Port Read1/1 -> NOT/1, B rise and A true/2, B fall and A true/2  "A true"
  Moving Forward/1 -> If/1
  Backward Value/1(dir) -> Merge/2
  B fall and A false/1 -> Moving Forward/2
  B rise and A true/1 -> Moving Forward/1
  Digital Port Read/1 -> Detect Decrease/1, Detect Increase/1
  Detect Decrease/1 -> B fall and A true/1, B fall and A false/1  "B fall"
  Forward Value/1(dir) -> Merge/1
  Moving Backward/1 -> If/2
  If/2 -> Backward Value/Action
  B fall and A true/1 -> Moving Backward/1
  If/1 -> Forward Value/Action
  Merge/1 -> dir/1
  B rise and A false/1 -> Moving Backward/2
  NOT/1 -> B rise and A false/2, B fall and A false/2  "A false"
  Detect Increase/1 -> B rise and A false/1, B rise and A true/1  "B rise"

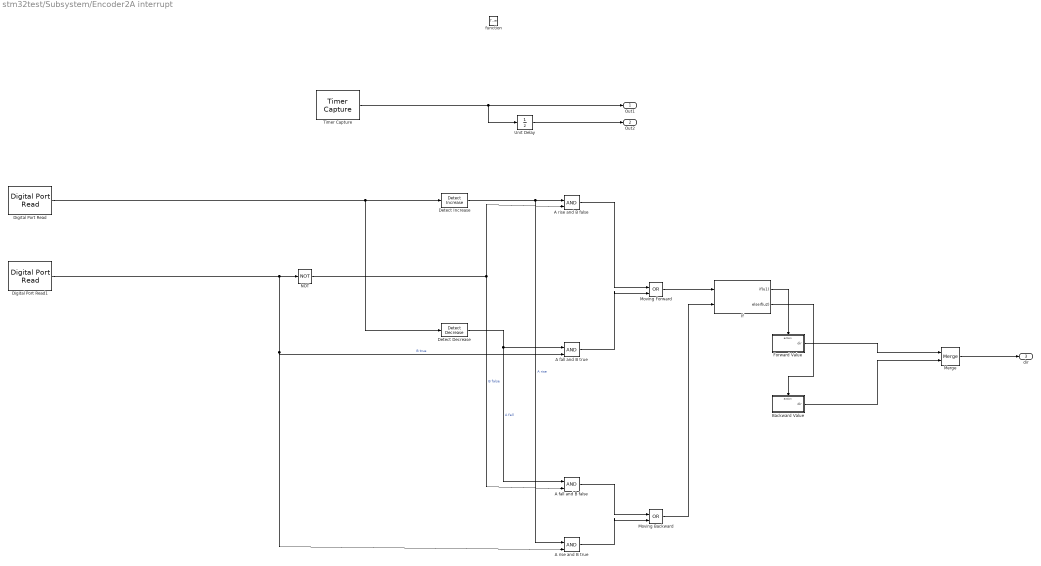
== system stm32test/Subsystem/Encoder2A interrupt ==
  function : TriggerPort  TriggerType=function-call  VariantControl=(inherit)
  A fall and B false : Logic  IconShape=distinctive  AllPortsSameDT=off  OutDataTypeStr=boolean
  A fall and B true : Logic  IconShape=distinctive  AllPortsSameDT=off  OutDataTypeStr=boolean
  A rise and B false : Logic  IconShape=distinctive  AllPortsSameDT=off  OutDataTypeStr=boolean
  A rise and B true : Logic  IconShape=distinctive  AllPortsSameDT=off  OutDataTypeStr=boolean
  Backward Value : Subsystem  TreatAsAtomicUnit=on
  Detect Decrease : simulink/Logic and Bit Operations/Detect Decrease  vinit=0.0  OutDataTypeStr=boolean
  Detect Increase : simulink/Logic and Bit Operations/Detect Increase  vinit=0.0  OutDataTypeStr=boolean
  Digital Port Read : stm32f4xxblockslib/Digital Port Read  PortName=GPIOA  PinNumber=[2]  ReadOperation=on  IOAsArray=on  SampleTime=-1  EnableSimPort=off  hoistedMaskSrc=ECSoC/ECSimCodegen/Digital Port Read
  Digital Port Read1 : stm32f4xxblockslib/Digital Port Read  PortName=GPIOA  PinNumber=[3]  ReadOperation=on  IOAsArray=on  SampleTime=-1  EnableSimPort=off  hoistedMaskSrc=ECSoC/ECSimCodegen/Digital Port Read
  Forward Value : Subsystem  TreatAsAtomicUnit=on
  If : If  NumInputs=2  IfExpression=u1  ElseIfExpressions=u2  ShowElse=off
  Merge : Merge
  Moving Backward : Logic  Operator=OR  IconShape=distinctive  AllPortsSameDT=off  OutDataTypeStr=boolean
  Moving Forward : Logic  Operator=OR  IconShape=distinctive  AllPortsSameDT=off  OutDataTypeStr=boolean
  NOT : Logic  Operator=NOT  IconShape=distinctive  AllPortsSameDT=off  OutDataTypeStr=boolean
  Timer Capture : stm32blockslib/Timer Capture  TimerModule=TIM5  SelectedChannel=CH3  CaptureLength=1  OutputDataLength=off  OutputOverrunStatus=off  OutputDirection=off  SampleTime=-1
      settings: LibrarySourceBlock=stm32f4xxblockslib/Timer Capture
  Unit Delay : UnitDelay  SampleTime=-1  HasFrameUpgradeWarning=on
  Out1 : Outport
  Out2 : Outport  Port=2
  dir : Outport  Port=3
  wires:
  Unit Delay/1 -> Out2/1
  If/1 -> Forward Value/Action
  If/2 -> Backward Value/Action
  A rise and B false/1 -> Moving Forward/1
  A fall and B false/1 -> Moving Backward/1
  Moving Forward/1 -> If/1
  A rise and B true/1 -> Moving Backward/2
  Forward Value/1(dir) -> Merge/1
  A fall and B true/1 -> Moving Forward/2
  Digital Port Read1/1 -> A rise and B true/2, A fall and B true/2, NOT/1  "B true"
  Merge/1 -> dir/1
  Detect Increase/1 -> A rise and B true/1, A rise and B false/1  "A rise"
  NOT/1 -> A fall and B false/2, A rise and B false/2  "B false"
  Moving Backward/1 -> If/2
  Detect Decrease/1 -> A fall and B false/1, A fall and B true/1  "A fall"
  Backward Value/1(dir) -> Merge/2
  Digital Port Read/1 -> Detect Increase/1, Detect Decrease/1
  Timer Capture/1 -> Unit Delay/1, Out1/1

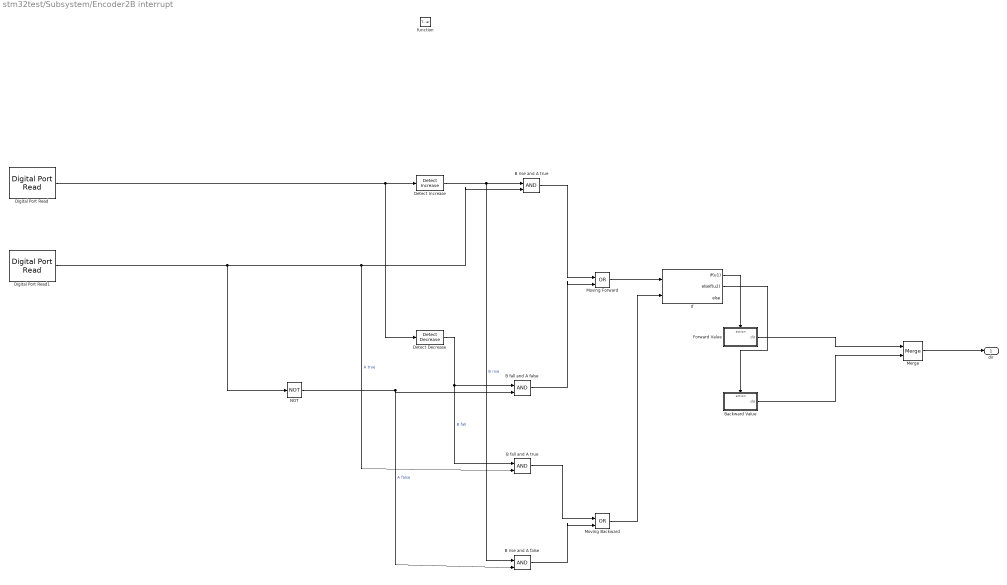
== system stm32test/Subsystem/Encoder2B interrupt ==
  function : TriggerPort  TriggerType=function-call  VariantControl=(inherit)
  B fall and A false : Logic  IconShape=distinctive  AllPortsSameDT=off  OutDataTypeStr=boolean
  B fall and A true : Logic  IconShape=distinctive  AllPortsSameDT=off  OutDataTypeStr=boolean
  B rise and A false : Logic  IconShape=distinctive  AllPortsSameDT=off  OutDataTypeStr=boolean
  B rise and A true : Logic  IconShape=distinctive  AllPortsSameDT=off  OutDataTypeStr=boolean
  Backward Value : Subsystem  TreatAsAtomicUnit=on
  Detect Decrease : simulink/Logic and Bit Operations/Detect Decrease  vinit=0.0  OutDataTypeStr=boolean
  Detect Increase : simulink/Logic and Bit Operations/Detect Increase  vinit=0.0  OutDataTypeStr=boolean
  Digital Port Read : stm32f4xxblockslib/Digital Port Read  PortName=GPIOA  PinNumber=[3]  ReadOperation=on  IOAsArray=on  SampleTime=-1  EnableSimPort=off  hoistedMaskSrc=ECSoC/ECSimCodegen/Digital Port Read
  Digital Port Read1 : stm32f4xxblockslib/Digital Port Read  PortName=GPIOA  PinNumber=[2]  ReadOperation=on  IOAsArray=on  SampleTime=-1  EnableSimPort=off  hoistedMaskSrc=ECSoC/ECSimCodegen/Digital Port Read
  Forward Value : Subsystem  TreatAsAtomicUnit=on
  If : If  NumInputs=2  IfExpression=u1  ElseIfExpressions=u2
  Merge : Merge
  Moving Backward : Logic  Operator=OR  IconShape=distinctive  AllPortsSameDT=off  OutDataTypeStr=boolean
  Moving Forward : Logic  Operator=OR  IconShape=distinctive  AllPortsSameDT=off  OutDataTypeStr=boolean
  NOT : Logic  Operator=NOT  IconShape=distinctive  AllPortsSameDT=off  OutDataTypeStr=boolean
  dir : Outport
  wires:
  Backward Value/1(dir) -> Merge/2
  Forward Value/1(dir) -> Merge/1
  If/2 -> Backward Value/Action
  If/1 -> Forward Value/Action
  Merge/1 -> dir/1
  Digital Port Read1/1 -> NOT/1, B rise and A true/2, B fall and A true/2  "A true"
  B rise and A false/1 -> Moving Backward/2
  Detect Decrease/1 -> B fall and A true/1, B fall and A false/1  "B fall"
  B fall and A true/1 -> Moving Backward/1
  Moving Forward/1 -> If/1
  NOT/1 -> B rise and A false/2, B fall and A false/2  "A false"
  Moving Backward/1 -> If/2
  B rise and A true/1 -> Moving Forward/1
  B fall and A false/1 -> Moving Forward/2
  Digital Port Read/1 -> Detect Decrease/1, Detect Increase/1
  Detect Increase/1 -> B rise and A false/1, B rise and A true/1  "B rise"

== system stm32test/Subsystem/Moving1 ==
  omega : Inport
  Action Port : ActionPort  ActionPortLabel=else
  Out1 : Outport
  wires:
  omega/1 -> Out1/1

== system stm32test/Subsystem/Moving2 ==
  In1 : Inport
  Action Port : ActionPort  ActionPortLabel=else
  Out1 : Outport
  wires:
  In1/1 -> Out1/1

== system stm32test/Subsystem/Stopped1 ==
  Action Port : ActionPort  ActionPortLabel=if(u1)
  Constant : Constant  Value=0
  Out1 : Outport
  wires:
  Constant/1 -> Out1/1

== system stm32test/Subsystem/Stopped2 ==
  Action Port : ActionPort  ActionPortLabel=if(u1)
  Constant : Constant  Value=0
  Out1 : Outport
  wires:
  Constant/1 -> Out1/1

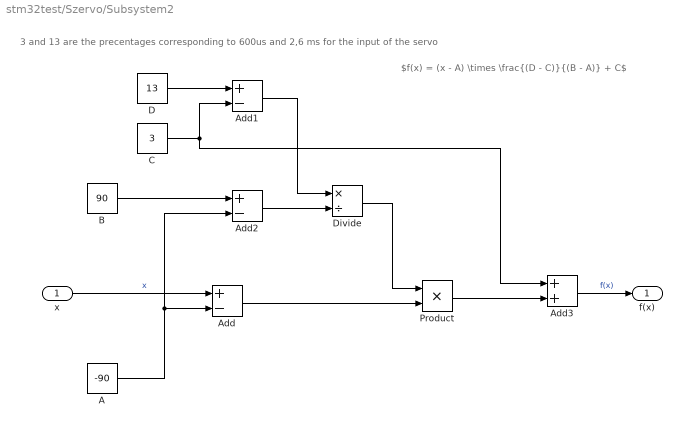
== system stm32test/Szervo/Subsystem2 ==
  note: 3 and 13 are the precentages corresponding to 600us and 2,6 ms for the input of the servo
  note: $f(x) = (x - A) \times \frac{(D - C)}{(B - A)} + C$
  x : Inport
  A : Constant  Value=-90
  Add : Sum  Inputs=+-
  Add1 : Sum  Inputs=+-
  Add2 : Sum  Inputs=+-
  Add3 : Sum
  B : Constant  Value=90
  C : Constant  Value=3
  D : Constant  Value=13
  Divide : Product  Inputs=*/
  Product : Product
  f(x) : Outport
  wires:
  x/1 -> Add/1  "x"
  A/1 -> Add2/2, Add/2
  Add/1 -> Product/2
  D/1 -> Add1/1
  C/1 -> Add1/2, Add3/1
  Add1/1 -> Divide/1
  Add2/1 -> Divide/2
  B/1 -> Add2/1
  Product/1 -> Add3/2
  Add3/1 -> f(x)/1  "f(x)"
  Divide/1 -> Product/1

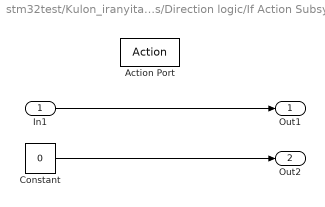
== system stm32test/Kulon_iranyitas/Direction logic/If Action Subsystem ==
  In1 : Inport
  Action Port : ActionPort  ActionPortLabel=else
  Constant : Constant  Value=0
  Out1 : Outport
  Out2 : Outport  Port=2
  wires:
  In1/1 -> Out1/1
  Constant/1 -> Out2/1

== system stm32test/Kulon_iranyitas/Direction logic/If Action Subsystem1 ==
  In1 : Inport
  Action Port : ActionPort  ActionPortLabel=if(u1)
  Constant : Constant  Value=0
  Out1 : Outport
  Out2 : Outport  Port=2
  wires:
  In1/1 -> Out1/1
  Constant/1 -> Out2/1

== system stm32test/Kulon_iranyitas/Direction logic/If Action Subsystem2 ==
  In1 : Inport
  Action Port : ActionPort  ActionPortLabel=if(u1)
  Constant : Constant  Value=0
  Out1 : Outport
  Out2 : Outport  Port=2
  wires:
  In1/1 -> Out1/1
  Constant/1 -> Out2/1

== system stm32test/Kulon_iranyitas/Direction logic/If Action Subsystem3 ==
  In1 : Inport
  Action Port : ActionPort  ActionPortLabel=else
  Constant : Constant  Value=0
  Out1 : Outport
  Out2 : Outport  Port=2
  wires:
  In1/1 -> Out1/1
  Constant/1 -> Out2/1

== system stm32test/Subsystem/Encoder1A interrupt/Backward Value ==
  Action Port : ActionPort  ActionPortLabel=elseif(u2)
  Constant : Constant  Value=bckvalue1
  dir : Outport
  wires:
  Constant/1 -> dir/1

== system stm32test/Subsystem/Encoder1A interrupt/Forward Value ==
  Action Port : ActionPort  ActionPortLabel=if(u1)
  Constant : Constant  Value=fwdvalue1
  dir : Outport
  wires:
  Constant/1 -> dir/1

== system stm32test/Subsystem/Encoder1B interrupt/Backward Value ==
  Action Port : ActionPort  ActionPortLabel=elseif(u2)
  Constant : Constant  Value=bckvalue1
  dir : Outport
  wires:
  Constant/1 -> dir/1

== system stm32test/Subsystem/Encoder1B interrupt/Forward Value ==
  Action Port : ActionPort  ActionPortLabel=if(u1)
  Constant : Constant  Value=fwdvalue1
  dir : Outport
  wires:
  Constant/1 -> dir/1

== system stm32test/Subsystem/Encoder2A interrupt/Backward Value ==
  Action Port : ActionPort  ActionPortLabel=elseif(u2)
  Constant : Constant  Value=bckvalue2
  dir : Outport
  wires:
  Constant/1 -> dir/1

== system stm32test/Subsystem/Encoder2A interrupt/Forward Value ==
  Action Port : ActionPort  ActionPortLabel=if(u1)
  Constant : Constant  Value=fwdvalue2
  dir : Outport
  wires:
  Constant/1 -> dir/1

== system stm32test/Subsystem/Encoder2B interrupt/Backward Value ==
  Action Port : ActionPort  ActionPortLabel=elseif(u2)
  Constant : Constant  Value=bckvalue2
  dir : Outport
  wires:
  Constant/1 -> dir/1

== system stm32test/Subsystem/Encoder2B interrupt/Forward Value ==
  Action Port : ActionPort  ActionPortLabel=if(u1)
  Constant : Constant  Value=fwdvalue2
  dir : Outport
  wires:
  Constant/1 -> dir/1
